simulink model "aero_forces"  (Simulink 7.5)
settings: Solver=ode45  StartTime=0.0  StopTime=10.0  RelTol=1e-3
values from neighbouring files (symbols this model uses):
  CL2 = -Cdcg*Sg*Lgz    (= -1.344)    [valuables.m]
  CM1 = K21*Nk*Sh*I2*L    (= 217.968531349)    [valuables.m]
  CM2 = (-1/2)*DiffCLAlpha*Sf*Nf*Lf1    (= -59.34811401)    [valuables.m]
  CM3 = -((Cdch*J2*Sh*L)+(Cdcf*Sf*Lf2))    (= -168.6714915)    [valuables.m]
  CX1 = -(Cdh0*Sh+Cdf0*Sf+Cdg0*Sg)    (= -0.6313245)    [valuables.m]
  CY1 = K21*Nk*Sh*I1    (= -6.9497212894)    [valuables.m]
  CY2 = (-1/2)*DiffCLAlpha*Sf*Nf    (= -8.4181722)    [valuables.m]
  CY3 = -((Cdch*J1*Sh)+(Cdcf*Sf)+(Cdcg*Sg))    (= -25.4932315)    [valuables.m]
  CZ3 = -((Cdch*J1*Sh)+(Cdcf*Sf))    (= -24.9332315)    [valuables.m]
undefined symbols (not defined in the file or in its folder): row, V
settings Model: Creator=knightofaccess  LastModifiedBy=knightofaccess

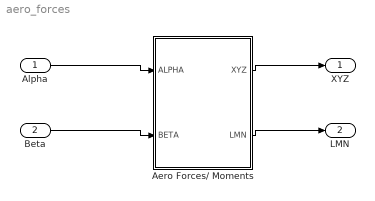
== system aero_forces ==
  Alpha : Inport  OutDataType=sfix(16)  OutScaling=2^0
  Beta : Inport  Port=2  OutDataType=sfix(16)  OutScaling=2^0
  Aero Forces/ Moments : Subsystem
  XYZ : Outport  OutDataType=sfix(16)  OutScaling=2^0
  LMN : Outport  Port=2  OutDataType=sfix(16)  OutScaling=2^0
  wires:
  Aero Forces/ Moments/1(XYZ) -> XYZ/1
  Aero Forces/ Moments/2(LMN) -> LMN/1
  Alpha/1 -> Aero Forces/ Moments/1(ALPHA)
  Beta/1 -> Aero Forces/ Moments/2(BETA)

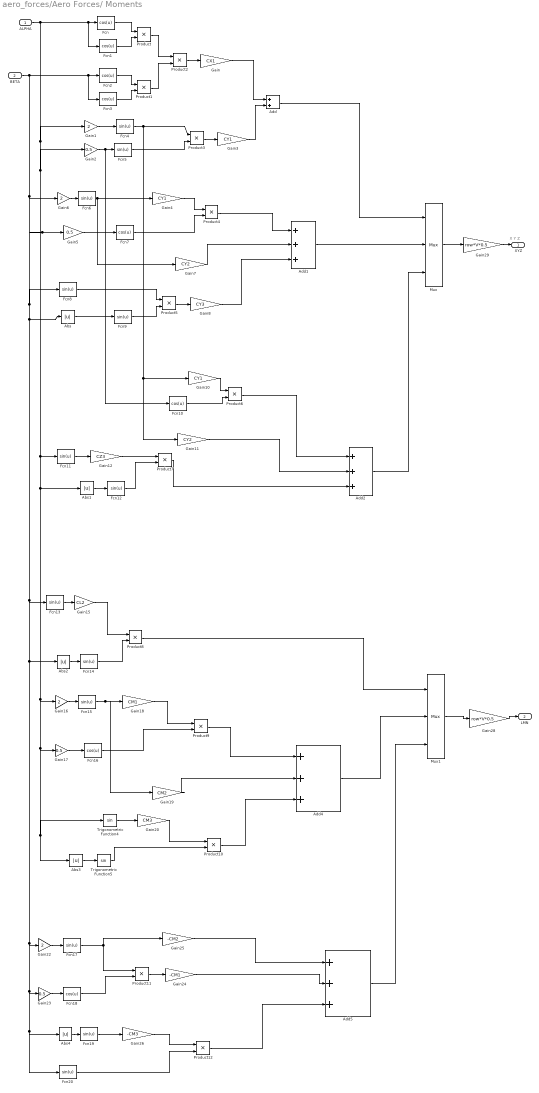
== system aero_forces/Aero Forces/ Moments ==
  note: X Y Z
  ALPHA : Inport  OutDataType=sfix(16)  OutScaling=2^0
  BETA : Inport  Port=2  OutDataType=sfix(16)  OutScaling=2^0
  Abs{,1..4} (5 alike) : Abs
  Add : Sum  OutDataType=sfix(16)  OutScaling=2^-10
  Add{1..2,4..5} (4 alike) : Sum  Inputs=+++  OutDataType=sfix(16)  OutScaling=2^-10
  Fcn{,1..3,7,10,16,18} (8 alike) : Fcn  Expr=cos(u)
  Fcn{4..6,8..9,11..15,17,19..20} (13 alike) : Fcn  Expr=sin(u)
  Gain : Gain  Gain=CX1  ParameterDataType=sfix(16)  ParameterScaling=2^0  OutDataType=sfix(16)  OutScaling=2^0
  Gain{1,6,16,22} (4 alike) : Gain  Gain=2  ParameterDataType=sfix(16)  ParameterScaling=2^0  OutDataType=sfix(16)  OutScaling=2^0
  Gain10 : Gain  Gain=CY1  ParameterDataType=sfix(16)  ParameterScaling=2^0  OutDataType=sfix(16)  OutScaling=2^0
  Gain11 : Gain  Gain=CY2  ParameterDataType=sfix(16)  ParameterScaling=2^0  OutDataType=sfix(16)  OutScaling=2^0
  Gain12 : Gain  Gain=CZ3  ParameterDataType=sfix(16)  ParameterScaling=2^0  OutDataType=sfix(16)  OutScaling=2^0
  Gain15 : Gain  Gain=CL2  ParameterDataType=sfix(16)  ParameterScaling=2^0  OutDataType=sfix(16)  OutScaling=2^0
  Gain{2,5,17,23} (4 alike) : Gain  Gain=0.5  ParameterDataType=sfix(16)  ParameterScaling=2^0  OutDataType=sfix(16)  OutScaling=2^0
  Gain18 : Gain  Gain=CM1  ParameterDataType=sfix(16)  ParameterScaling=2^0  OutDataType=sfix(16)  OutScaling=2^0
  Gain19 : Gain  Gain=CM2  ParameterDataType=sfix(16)  ParameterScaling=2^0  OutDataType=sfix(16)  OutScaling=2^0
  Gain20 : Gain  Gain=CM3  ParameterDataType=sfix(16)  ParameterScaling=2^0  OutDataType=sfix(16)  OutScaling=2^0
  Gain24 : Gain  Gain=-CM1  ParameterDataType=sfix(16)  ParameterScaling=2^0  OutDataType=sfix(16)  OutScaling=2^0
  Gain25 : Gain  Gain=-CM2  ParameterDataType=sfix(16)  ParameterScaling=2^0  OutDataType=sfix(16)  OutScaling=2^0
  Gain26 : Gain  Gain=-CM3  ParameterDataType=sfix(16)  ParameterScaling=2^0  OutDataType=sfix(16)  OutScaling=2^0
  Gain28 : Gain  Gain=row*V*0.5  ParameterDataType=sfix(16)  ParameterScaling=2^0  OutDataType=sfix(16)  OutScaling=2^0
  Gain29 : Gain  Gain=row*V*0.5  ParameterDataType=sfix(16)  ParameterScaling=2^0  OutDataType=sfix(16)  OutScaling=2^0
  Gain3 : Gain  Gain=CY1  ParameterDataType=sfix(16)  ParameterScaling=2^0  OutDataType=sfix(16)  OutScaling=2^0
  Gain4 : Gain  Gain=CY1  ParameterDataType=sfix(16)  ParameterScaling=2^0  OutDataType=sfix(16)  OutScaling=2^0
  Gain7 : Gain  Gain=CY2  ParameterDataType=sfix(16)  ParameterScaling=2^0  OutDataType=sfix(16)  OutScaling=2^0
  Gain8 : Gain  Gain=CY3  ParameterDataType=sfix(16)  ParameterScaling=2^0  OutDataType=sfix(16)  OutScaling=2^0
  Mux : Mux  Inputs=3
  Mux1 : Mux  Inputs=3
  Product{,1..12} (13 alike) : Product  OutDataType=sfix(16)  OutScaling=2^0  RndMeth=Zero
  Trigonometric Function4 : Trigonometry
  Trigonometric Function5 : Trigonometry
  XYZ : Outport  OutDataType=sfix(16)  OutScaling=2^0
  LMN : Outport  Port=2  OutDataType=sfix(16)  OutScaling=2^0
  wires:
  Mux1/1 -> Gain28/1
  Mux/1 -> Gain29/1
  Add5/1 -> Mux1/3
  Add4/1 -> Mux1/2
  Product12/1 -> Add5/3
  Gain24/1 -> Add5/2
  Gain25/1 -> Add5/1
  Gain26/1 -> Product12/1
  Fcn20/1 -> Product12/2
  Fcn19/1 -> Gain26/1
  Abs4/1 -> Fcn19/1
  Product11/1 -> Gain24/1
  Fcn18/1 -> Product11/2
  Gain23/1 -> Fcn18/1
  Fcn17/1 -> Product11/1, Gain25/1
  Gain22/1 -> Fcn17/1
  Product10/1 -> Add4/3
  Gain19/1 -> Add4/2
  Product9/1 -> Add4/1
  Gain20/1 -> Product10/1
  Trigonometric Function4/1 -> Gain20/1
  Trigonometric Function5/1 -> Product10/2
  Abs3/1 -> Trigonometric Function5/1
  Gain18/1 -> Product9/1
  Fcn16/1 -> Product9/2
  Fcn15/1 -> Gain18/1, Gain19/1
  Gain17/1 -> Fcn16/1
  Gain16/1 -> Fcn15/1
  Product8/1 -> Mux1/1
  Fcn14/1 -> Product8/2
  Gain15/1 -> Product8/1
  Abs2/1 -> Fcn14/1
  Fcn13/1 -> Gain15/1
  Add2/1 -> Mux/3
  Add1/1 -> Mux/2
  Add/1 -> Mux/1
  Product7/1 -> Add2/3
  Gain11/1 -> Add2/2
  Product6/1 -> Add2/1
  Fcn12/1 -> Product7/2
  Abs1/1 -> Fcn12/1
  Fcn10/1 -> Product6/2
  Gain10/1 -> Product6/1
  Gain8/1 -> Add1/3
  Gain7/1 -> Add1/2
  Product4/1 -> Add1/1
  Product5/1 -> Gain8/1
  Fcn9/1 -> Product5/2
  Fcn8/1 -> Product5/1
  Abs/1 -> Fcn9/1
  Gain4/1 -> Product4/1
  Fcn7/1 -> Product4/2
  Gain6/1 -> Fcn6/1
  Fcn6/1 -> Gain4/1, Gain7/1
  Gain5/1 -> Fcn7/1
  Gain3/1 -> Add/2
  Gain/1 -> Add/1
  Product3/1 -> Gain3/1
  Fcn5/1 -> Product3/2
  Fcn4/1 -> Product3/1, Gain10/1, Gain11/1
  Gain2/1 -> Fcn5/1, Fcn10/1
  Gain1/1 -> Fcn4/1
  Product2/1 -> Gain/1
  Product1/1 -> Product2/2
  Product/1 -> Product2/1
  Fcn3/1 -> Product1/2
  Fcn2/1 -> Product1/1
  BETA/1 -> Fcn2/1, Fcn3/1, Gain6/1, Gain5/1, Abs/1, Abs2/1, Gain22/1, Gain23/1, Abs4/1, Fcn20/1, Fcn13/1, Fcn8/1
  Fcn1/1 -> Product/2
  Fcn/1 -> Product/1
  ALPHA/1 -> Fcn/1, Fcn1/1, Gain1/1, Gain2/1, Abs1/1, Gain16/1, Gain17/1, Trigonometric Function4/1, Abs3/1, Fcn11/1
  Gain29/1 -> XYZ/1
  Gain28/1 -> LMN/1
  Fcn11/1 -> Gain12/1
  Gain12/1 -> Product7/1
